simulink model "APSA"  (R2014b)
settings: Solver=FixedStepDiscrete  StartTime=0.0  StopTime=180  FixedStep=0.01  RelTol=1e-3
PreLoadFcn:
  | if exist('tl_preloadfcn','file'), tl_preloadfcn(gcs,400); end
PostLoadFcn:
  | if exist('tl_postloadfcn','file'), tl_postloadfcn(gcs,400); end
InitFcn:
  | if exist('tlds_init','file'), tlds_init(gcs); end
StartFcn:
  | if exist('tlds_start','file'), tlds_start(gcs); end
StopFcn:
  | if exist('tlds_stop','file'), tlds_stop(gcs); end
values from neighbouring files (symbols this model uses):
  EERAM_Map_Backward_Values = EERAM_Current_Map_Backward.signals.values(row,:)    [Create_Map.m]    (also in EERAM_Map_Backward_Values_2.mat = [0 0 0 0 0 0 150 150 150 150 150 150 ... (100 elements, 1x10)
  EERAM_Map_Forward_Values = EERAM_Current_Map_Forward.signals.values(row,:)    [Create_Map.m]    (also in EERAM_Map_Forward_Values_2.mat = [150 150 150 150 150 150 150 150 150 150 150 150 ... (100 el)
undefined symbols (not defined in the file or in its folder): sigbuilder_block
libraries: tllib x2
(part 2 of 3)

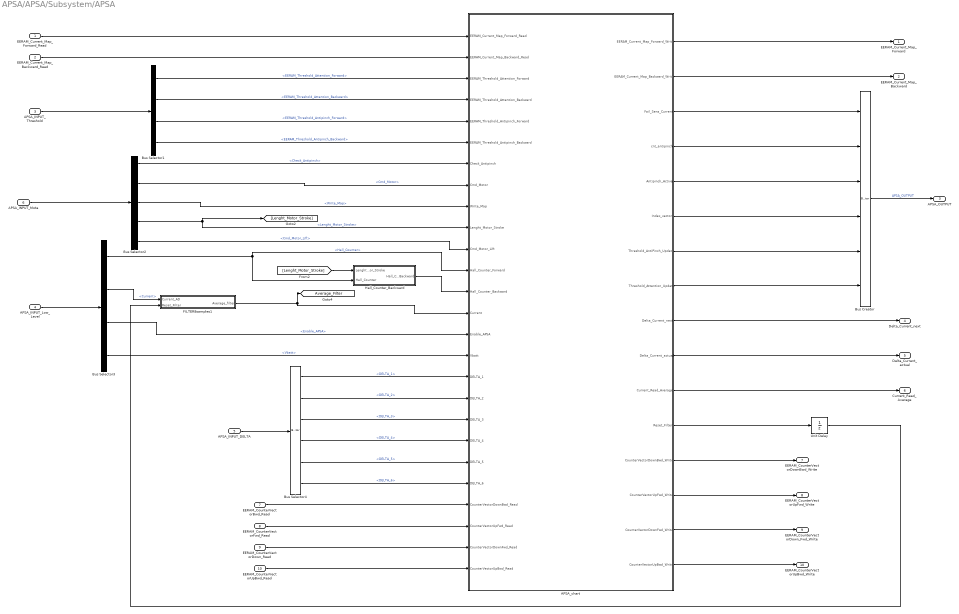
== system APSA/APSA/Subsystem/APSA ==
  EERAM_Current_Map_Forward_Read : Inport  PortDimensions=100  mask(TL_Inport){data={'output',{'variable','EERAM_Current_Map_Forward'},'date',736223.65085809026}}
      settings: DeleteFcn=if exist('delete_tlblock','file')==2,delete_tlblock(gcbh);end  OpenFcn=if exist('tl_open_blockdlg','file')==2,tl_open_blockdlg(gcbh);else,open_system(gcbh,'parameter');end
      settings: CopyFcn=|
      | if exist('tl_reset_reviewflag','file')==2
      |     tl_reset_reviewflag(gcbh);
      | end
      | if exist('tl_check_ports','file')
      |     tl_check_ports(gcbh);
      | end
      settings: NameChangeFcn=|
      | if exist('rename_tlblock','file')==2,rename_tlblock(gcbh);end
      | if exist('tl_check_ports','file'), tl_check_ports(gcbh); end
      mask Help: eval(['if exist(''tl_online_help'',''file'') == 2, tl_online_help(''Topic'',''TL_Inport''),else, web([''jar:file:///'',matlabroot,''/help/toolbox/simulink/help.jar!/slref/' lower(get_param(gcbh,'Blocktype')) '.html''], ''-helpbrowser''),end'])
      mask Display: plot([0.2 0.35 NaN 0.65 0.8],[0 1 NaN 0 1]);
  EERAM_Current_Map_Backward_Read : Inport  Port=2  PortDimensions=100  mask(TL_Inport){data={'output',{'variable','EERAM_Current_Map_Backward'},'date',736223.65094585647}}
      settings: DeleteFcn=if exist('delete_tlblock','file')==2,delete_tlblock(gcbh);end  OpenFcn=if exist('tl_open_blockdlg','file')==2,tl_open_blockdlg(gcbh);else,open_system(gcbh,'parameter');end
      settings: CopyFcn=|
      | if exist('tl_reset_reviewflag','file')==2
      |     tl_reset_reviewflag(gcbh);
      | end
      | if exist('tl_check_ports','file')
      |     tl_check_ports(gcbh);
      | end
      settings: NameChangeFcn=|
      | if exist('rename_tlblock','file')==2,rename_tlblock(gcbh);end
      | if exist('tl_check_ports','file'), tl_check_ports(gcbh); end
      mask Help: eval(['if exist(''tl_online_help'',''file'') == 2, tl_online_help(''Topic'',''TL_Inport''),else, web([''jar:file:///'',matlabroot,''/help/toolbox/simulink/help.jar!/slref/' lower(get_param(gcbh,'Blocktype')) '.html''], ''-helpbrowser''),end'])
      mask Display: plot([0.2 0.35 NaN 0.65 0.8],[0 1 NaN 0 1]);
  APSA_INPUT_Threshold : Inport  Port=3  mask(TL_BusInport){data={'#autoscaling',4,'#message',4,'#output',4,'#logdata',4,'output#1',{'variable','EERAM_Threshold_Att_Forward'},'output#2',{'variable','EERAM_Threshold_Att_Backward'},'output#3',{'variable','EERAM_Threshold_Antipinch_Forward'},'output#4',{'variable','EERAM_Threshold_Antipinch_Backward'},'signals',{{'APSA_INPUT_Threshold',{'EERAM_Threshold_Attention_Forward';'EERAM_Threshold_Attention_Backward';'EERAM_Threshold_Antipinch_Forward';'EERAM_Threshold_Antipinch_Backward'}}},'date',736307.73504877312}}
      settings: DeleteFcn=if exist('delete_tlblock','file')==2,delete_tlblock(gcbh);end  OpenFcn=if exist('tl_open_blockdlg','file')==2,tl_open_blockdlg(gcbh);else,open_system(gcbh,'parameter');end
      settings: CopyFcn=|
      | if exist('tl_reset_reviewflag','file')==2
      |     tl_reset_reviewflag(gcbh);
      | end
      | if exist('tl_check_ports','file')
      |     tl_check_ports(gcbh);
      | end
      settings: NameChangeFcn=|
      | if exist('rename_tlblock','file')==2,rename_tlblock(gcbh);end
      | if exist('tl_check_ports','file'), tl_check_ports(gcbh); end
      mask Help: eval(['if exist(''tl_online_help'',''file'') == 2, tl_online_help(''Topic'',''TL_Inport''),else, web([''jar:file:///'',matlabroot,''/help/toolbox/simulink/help.jar!/slref/' lower(get_param(gcbh,'Blocktype')) '.html''], ''-helpbrowser''),end'])
      mask Display: plot([0.2 0.35 NaN 0.65 0.8],[0 1 NaN 0 1]);
  APSA_INPUT_Low_Level : Inport  Port=4  mask(TL_BusInport){data={'#autoscaling',4,'#message',4,'#output',4,'#logdata',4,'output#1',{'name','$L','max',10000,'min',-10000},'output#2',{'name','$L','type','UInt16'},'output#3',{'name','$L','type','UInt8'},'output#4',{'name','$L'},'structvar',{'type','IMPLICIT_STRUCT','name','$L'},'signals',{{'APSA_INPUT_Low_Level',{'Hall_Counter';'Current';'Enable_APSA';'Vbatt'}}},'date',736393.5789320023}}
      settings: DeleteFcn=if exist('delete_tlblock','file')==2,delete_tlblock(gcbh);end  OpenFcn=if exist('tl_open_blockdlg','file')==2,tl_open_blockdlg(gcbh);else,open_system(gcbh,'parameter');end
      settings: CopyFcn=|
      | if exist('tl_reset_reviewflag','file')==2
      |     tl_reset_reviewflag(gcbh);
      | end
      | if exist('tl_check_ports','file')
      |     tl_check_ports(gcbh);
      | end
      settings: NameChangeFcn=|
      | if exist('rename_tlblock','file')==2,rename_tlblock(gcbh);end
      | if exist('tl_check_ports','file'), tl_check_ports(gcbh); end
      mask Help: eval(['if exist(''tl_online_help'',''file'') == 2, tl_online_help(''Topic'',''TL_Inport''),else, web([''jar:file:///'',matlabroot,''/help/toolbox/simulink/help.jar!/slref/' lower(get_param(gcbh,'Blocktype')) '.html''], ''-helpbrowser''),end'])
      mask Display: plot([0.2 0.35 NaN 0.65 0.8],[0 1 NaN 0 1]);
  APSA_INPUT_DELTA : Inport  Port=5  mask(TL_BusInport){data={'#autoscaling',6,'#message',6,'#output',6,'#logdata',6,'output#1',{'name','$L','min',0,'type','UInt8'},'output#2',{'name','$L','min',0,'type','UInt8'},'output#3',{'name','$L','min',0,'type','UInt8'},'output#4',{'name','$L','min',0,'type','UInt8'},'output#5',{'name','$L','type','UInt8'},'output#6',{'name','$L','type','UInt8'},'structvar',{'type','IMPLICIT_STRUCT','name','$L'},'signals',{{'APSA_INPUT_DELTA',{'DELTA_1';'DELTA_2';'DELTA_3';'DELTA_4';'DELTA_5';'DELTA_6'}}},'date',736307.735760162}}
      settings: DeleteFcn=if exist('delete_tlblock','file')==2,delete_tlblock(gcbh);end  OpenFcn=if exist('tl_open_blockdlg','file')==2,tl_open_blockdlg(gcbh);else,open_system(gcbh,'parameter');end
      settings: CopyFcn=|
      | if exist('tl_reset_reviewflag','file')==2
      |     tl_reset_reviewflag(gcbh);
      | end
      | if exist('tl_check_ports','file')
      |     tl_check_ports(gcbh);
      | end
      settings: NameChangeFcn=|
      | if exist('rename_tlblock','file')==2,rename_tlblock(gcbh);end
      | if exist('tl_check_ports','file'), tl_check_ports(gcbh); end
      mask Help: eval(['if exist(''tl_online_help'',''file'') == 2, tl_online_help(''Topic'',''TL_Inport''),else, web([''jar:file:///'',matlabroot,''/help/toolbox/simulink/help.jar!/slref/' lower(get_param(gcbh,'Blocktype')) '.html''], ''-helpbrowser''),end'])
      mask Display: plot([0.2 0.35 NaN 0.65 0.8],[0 1 NaN 0 1]);
  APSA_INPUT_Mota : Inport  Port=6  mask(TL_BusInport){data={'#autoscaling',5,'#message',5,'#output',5,'#logdata',5,'output#1',{'name','$L','type','UInt8'},'output#2',{'name','$L','type','UInt8'},'output#3',{'name','$L','type','UInt8'},'output#4',{'name','$L','max',5000,'min',0,'type','UInt16'},'output#5',{'name','$L','type','UInt8'},'structvar',{'type','IMPLICIT_STRUCT','name','$L'},'signals',{{'APSA_INPUT_Mota',{'Cmd_Motor';'Write_Map';'Check_Antipinch';'Lenght_Motor_Stroke';'Cmd_Motor_Lift'}}},'date',736393.58703908569}}
      settings: DeleteFcn=if exist('delete_tlblock','file')==2,delete_tlblock(gcbh);end  OpenFcn=if exist('tl_open_blockdlg','file')==2,tl_open_blockdlg(gcbh);else,open_system(gcbh,'parameter');end
      settings: CopyFcn=|
      | if exist('tl_reset_reviewflag','file')==2
      |     tl_reset_reviewflag(gcbh);
      | end
      | if exist('tl_check_ports','file')
      |     tl_check_ports(gcbh);
      | end
      settings: NameChangeFcn=|
      | if exist('rename_tlblock','file')==2,rename_tlblock(gcbh);end
      | if exist('tl_check_ports','file'), tl_check_ports(gcbh); end
      mask Help: eval(['if exist(''tl_online_help'',''file'') == 2, tl_online_help(''Topic'',''TL_Inport''),else, web([''jar:file:///'',matlabroot,''/help/toolbox/simulink/help.jar!/slref/' lower(get_param(gcbh,'Blocktype')) '.html''], ''-helpbrowser''),end'])
      mask Display: plot([0.2 0.35 NaN 0.65 0.8],[0 1 NaN 0 1]);
  EERAM_CounterVectorBwd_Read : Inport  Port=7  PortDimensions=13  mask(TL_Inport){data={'output',{'variable','EERAM_CounterVectorDownBwd'},'date',736349.65360806708}}
      settings: DeleteFcn=if exist('delete_tlblock','file')==2,delete_tlblock(gcbh);end  OpenFcn=if exist('tl_open_blockdlg','file')==2,tl_open_blockdlg(gcbh);else,open_system(gcbh,'parameter');end
      settings: CopyFcn=|
      | if exist('tl_reset_reviewflag','file')==2
      |     tl_reset_reviewflag(gcbh);
      | end
      | if exist('tl_check_ports','file')
      |     tl_check_ports(gcbh);
      | end
      settings: NameChangeFcn=|
      | if exist('rename_tlblock','file')==2,rename_tlblock(gcbh);end
      | if exist('tl_check_ports','file'), tl_check_ports(gcbh); end
      mask Help: eval(['if exist(''tl_online_help'',''file'') == 2, tl_online_help(''Topic'',''TL_Inport''),else, web([''jar:file:///'',matlabroot,''/help/toolbox/simulink/help.jar!/slref/' lower(get_param(gcbh,'Blocktype')) '.html''], ''-helpbrowser''),end'])
      mask Display: plot([0.2 0.35 NaN 0.65 0.8],[0 1 NaN 0 1]);
  EERAM_CounterVectorFwd_Read : Inport  Port=8  PortDimensions=13  mask(TL_Inport){data={'output',{'variable','EERAM_CounterVectorUpFwd'},'date',736349.65366483794}}
      settings: DeleteFcn=if exist('delete_tlblock','file')==2,delete_tlblock(gcbh);end  OpenFcn=if exist('tl_open_blockdlg','file')==2,tl_open_blockdlg(gcbh);else,open_system(gcbh,'parameter');end
      settings: CopyFcn=|
      | if exist('tl_reset_reviewflag','file')==2
      |     tl_reset_reviewflag(gcbh);
      | end
      | if exist('tl_check_ports','file')
      |     tl_check_ports(gcbh);
      | end
      settings: NameChangeFcn=|
      | if exist('rename_tlblock','file')==2,rename_tlblock(gcbh);end
      | if exist('tl_check_ports','file'), tl_check_ports(gcbh); end
      mask Help: eval(['if exist(''tl_online_help'',''file'') == 2, tl_online_help(''Topic'',''TL_Inport''),else, web([''jar:file:///'',matlabroot,''/help/toolbox/simulink/help.jar!/slref/' lower(get_param(gcbh,'Blocktype')) '.html''], ''-helpbrowser''),end'])
      mask Display: plot([0.2 0.35 NaN 0.65 0.8],[0 1 NaN 0 1]);
  EERAM_CounterVectorDown_Read : Inport  Port=9  PortDimensions=13  mask(TL_Inport){data={'output',{'variable','EERAM_CounterVectorDownFwd'},'date',736349.6566348843}}
      settings: DeleteFcn=if exist('delete_tlblock','file')==2,delete_tlblock(gcbh);end  OpenFcn=if exist('tl_open_blockdlg','file')==2,tl_open_blockdlg(gcbh);else,open_system(gcbh,'parameter');end
      settings: CopyFcn=|
      | if exist('tl_reset_reviewflag','file')==2
      |     tl_reset_reviewflag(gcbh);
      | end
      | if exist('tl_check_ports','file')
      |     tl_check_ports(gcbh);
      | end
      settings: NameChangeFcn=|
      | if exist('rename_tlblock','file')==2,rename_tlblock(gcbh);end
      | if exist('tl_check_ports','file'), tl_check_ports(gcbh); end
      mask Help: eval(['if exist(''tl_online_help'',''file'') == 2, tl_online_help(''Topic'',''TL_Inport''),else, web([''jar:file:///'',matlabroot,''/help/toolbox/simulink/help.jar!/slref/' lower(get_param(gcbh,'Blocktype')) '.html''], ''-helpbrowser''),end'])
      mask Display: plot([0.2 0.35 NaN 0.65 0.8],[0 1 NaN 0 1]);
  EERAM_CounterVectorUpBwd_Read : Inport  Port=10  PortDimensions=13  mask(TL_Inport){data={'output',{'variable','EERAM_CounterVectorUpBwd'},'date',736349.6567374653}}
      settings: DeleteFcn=if exist('delete_tlblock','file')==2,delete_tlblock(gcbh);end  OpenFcn=if exist('tl_open_blockdlg','file')==2,tl_open_blockdlg(gcbh);else,open_system(gcbh,'parameter');end
      settings: CopyFcn=|
      | if exist('tl_reset_reviewflag','file')==2
      |     tl_reset_reviewflag(gcbh);
      | end
      | if exist('tl_check_ports','file')
      |     tl_check_ports(gcbh);
      | end
      settings: NameChangeFcn=|
      | if exist('rename_tlblock','file')==2,rename_tlblock(gcbh);end
      | if exist('tl_check_ports','file'), tl_check_ports(gcbh); end
      mask Help: eval(['if exist(''tl_online_help'',''file'') == 2, tl_online_help(''Topic'',''TL_Inport''),else, web([''jar:file:///'',matlabroot,''/help/toolbox/simulink/help.jar!/slref/' lower(get_param(gcbh,'Blocktype')) '.html''], ''-helpbrowser''),end'])
      mask Display: plot([0.2 0.35 NaN 0.65 0.8],[0 1 NaN 0 1]);
  APSA_chart : Stateflow chart  TreatAsAtomicUnit=on
  Bus Creator : BusCreator  Inputs=6
  Bus Selector1 : BusSelector  OutputSignals=EERAM_Threshold_Attention_Forward,EERAM_Threshold_Attention_Backward,EERAM_Threshold_Antipinch_Forward,EERAM_Threshold_Antipinch_Backward
  Bus Selector2 : BusSelector  OutputSignals=Check_Antipinch,Cmd_Motor,Write_Map,Lenght_Motor_Stroke,Cmd_Motor_Lift
  Bus Selector3 : BusSelector  OutputSignals=Hall_Counter,Current,Enable_APSA,Vbatt
  Bus Selector4 : BusSelector  OutputSignals=DELTA_1,DELTA_2,DELTA_3,DELTA_4,DELTA_5,DELTA_6
  FILTER8samples1 : Subsystem
  Hall_Counter_Backward : Subsystem
  Unit Delay : UnitDelay  SampleTime=-1  mask(TL_UnitDelay){data={'output',{'type','UInt8'},'state',{'type','UInt8'},'date',736291.48166902782}}
      settings: CopyFcn=if exist('tl_reset_reviewflag') == 2, tl_reset_reviewflag(gcbh); end  DeleteFcn=if exist('delete_tlblock','file')==2,delete_tlblock(gcbh);end  NameChangeFcn=if exist('rename_tlblock','file')==2,rename_tlblock(gcbh);end  OpenFcn=if exist('tl_open_blockdlg','file')==2,tl_open_blockdlg(gcbh);else,open_system(gcbh,'parameter');end
      mask Help: eval(['if exist(''tl_online_help'',''file'') == 2, tl_online_help(''Topic'',''TL_UnitDelay''),else, web([''jar:file:///'',matlabroot,''/help/toolbox/simulink/help.jar!/slref/' lower(get_param(gcbh,'Blocktype')) '.html''], ''-helpbrowser''),end'])
      mask Display: plot([-0.1, 1.05, NaN, -0.1, 1.05],[.01, .01, NaN, .99, .99]);
  EERAM_Current_Map_Forward : Outport  PortDimensions=100  mask(TL_Outport){data={'output',{'variable','EERAM_Current_Map_Forward'},'date',736223.65313251154}}
      settings: DeleteFcn=if exist('delete_tlblock','file')==2,delete_tlblock(gcbh);end  OpenFcn=if exist('tl_open_blockdlg','file')==2,tl_open_blockdlg(gcbh);else,open_system(gcbh,'parameter');end
      settings: CopyFcn=|
      | if exist('tl_reset_reviewflag','file')==2
      |     tl_reset_reviewflag(gcbh);
      | end
      | if exist('tl_check_ports','file')
      |     tl_check_ports(gcbh);
      | end
      settings: NameChangeFcn=|
      | if exist('rename_tlblock','file')==2,rename_tlblock(gcbh);end
      | if exist('tl_check_ports','file'), tl_check_ports(gcbh); end
      mask Help: eval(['if exist(''tl_online_help'',''file'') == 2, tl_online_help(''Topic'',''TL_Outport''),else, web([''jar:file:///'',matlabroot,''/help/toolbox/simulink/help.jar!/slref/' lower(get_param(gcbh,'Blocktype')) '.html''], ''-helpbrowser''),end'])
      mask Display: plot([0.2 0.35 NaN 0.65 0.8],[0 1 NaN 0 1]);
  EERAM_Current_Map_Backward : Outport  Port=2  PortDimensions=100  mask(TL_Outport){data={'output',{'variable','EERAM_Current_Map_Backward'},'date',736223.65323016199}}
      settings: DeleteFcn=if exist('delete_tlblock','file')==2,delete_tlblock(gcbh);end  OpenFcn=if exist('tl_open_blockdlg','file')==2,tl_open_blockdlg(gcbh);else,open_system(gcbh,'parameter');end
      settings: CopyFcn=|
      | if exist('tl_reset_reviewflag','file')==2
      |     tl_reset_reviewflag(gcbh);
      | end
      | if exist('tl_check_ports','file')
      |     tl_check_ports(gcbh);
      | end
      settings: NameChangeFcn=|
      | if exist('rename_tlblock','file')==2,rename_tlblock(gcbh);end
      | if exist('tl_check_ports','file'), tl_check_ports(gcbh); end
      mask Help: eval(['if exist(''tl_online_help'',''file'') == 2, tl_online_help(''Topic'',''TL_Outport''),else, web([''jar:file:///'',matlabroot,''/help/toolbox/simulink/help.jar!/slref/' lower(get_param(gcbh,'Blocktype')) '.html''], ''-helpbrowser''),end'])
      mask Display: plot([0.2 0.35 NaN 0.65 0.8],[0 1 NaN 0 1]);
  APSA_OUTPUT : Outport  Port=3  mask(TL_BusOutport){data={'#autoscaling',6,'#message',6,'#output',6,'#logdata',6,'output#1',{'variable','Fail_Sens_Current'},'output#2',{'name','$L'},'output#3',{'variable','Antipinch_Active'},'output#4',{'variable','Index_vector'},'output#5',{'variable','Threshold_AntiPinch_Update'},'output#6',{'variable','Threshold_Attention_Update'},'structvar',{'type','IMPLICIT_STRUCT','name','$L'},'signals',{{'APSA_OUTPUT',{'Fail_Sens_Current';'cnt_antipinch';'Antipinch_Active';'Index_vector';'Threshold_AntiPinch_Update';'Threshold_Attention_Update'}}},'date',736307.74256392359}}
      settings: DeleteFcn=if exist('delete_tlblock','file')==2,delete_tlblock(gcbh);end  OpenFcn=if exist('tl_open_blockdlg','file')==2,tl_open_blockdlg(gcbh);else,open_system(gcbh,'parameter');end
      settings: CopyFcn=|
      | if exist('tl_reset_reviewflag','file')==2
      |     tl_reset_reviewflag(gcbh);
      | end
      | if exist('tl_check_ports','file')
      |     tl_check_ports(gcbh);
      | end
      settings: NameChangeFcn=|
      | if exist('rename_tlblock','file')==2,rename_tlblock(gcbh);end
      | if exist('tl_check_ports','file'), tl_check_ports(gcbh); end
      mask Help: eval(['if exist(''tl_online_help'',''file'') == 2, tl_online_help(''Topic'',''TL_Outport''),else, web([''jar:file:///'',matlabroot,''/help/toolbox/simulink/help.jar!/slref/' lower(get_param(gcbh,'Blocktype')) '.html''], ''-helpbrowser''),end'])
      mask Display: plot([0.2 0.35 NaN 0.65 0.8],[0 1 NaN 0 1]);
  Delta_Current_next : Outport  Port=4  mask(TL_Outport){data={'output',{'name','Delta_Current_next'},'date',736293.39429296297}}
      settings: DeleteFcn=if exist('delete_tlblock','file')==2,delete_tlblock(gcbh);end  OpenFcn=if exist('tl_open_blockdlg','file')==2,tl_open_blockdlg(gcbh);else,open_system(gcbh,'parameter');end
      settings: CopyFcn=|
      | if exist('tl_reset_reviewflag','file')==2
      |     tl_reset_reviewflag(gcbh);
      | end
      | if exist('tl_check_ports','file')
      |     tl_check_ports(gcbh);
      | end
      settings: NameChangeFcn=|
      | if exist('rename_tlblock','file')==2,rename_tlblock(gcbh);end
      | if exist('tl_check_ports','file'), tl_check_ports(gcbh); end
      mask Help: eval(['if exist(''tl_online_help'',''file'') == 2, tl_online_help(''Topic'',''TL_Outport''),else, web([''jar:file:///'',matlabroot,''/help/toolbox/simulink/help.jar!/slref/' lower(get_param(gcbh,'Blocktype')) '.html''], ''-helpbrowser''),end'])
      mask Display: plot([0.2 0.35 NaN 0.65 0.8],[0 1 NaN 0 1]);
  Delta_Current_actual : Outport  Port=5  mask(TL_Outport){data={'output',{'name','Delta_Current_actual'},'date',736293.39420129627}}
      settings: DeleteFcn=if exist('delete_tlblock','file')==2,delete_tlblock(gcbh);end  OpenFcn=if exist('tl_open_blockdlg','file')==2,tl_open_blockdlg(gcbh);else,open_system(gcbh,'parameter');end
      settings: CopyFcn=|
      | if exist('tl_reset_reviewflag','file')==2
      |     tl_reset_reviewflag(gcbh);
      | end
      | if exist('tl_check_ports','file')
      |     tl_check_ports(gcbh);
      | end
      settings: NameChangeFcn=|
      | if exist('rename_tlblock','file')==2,rename_tlblock(gcbh);end
      | if exist('tl_check_ports','file'), tl_check_ports(gcbh); end
      mask Help: eval(['if exist(''tl_online_help'',''file'') == 2, tl_online_help(''Topic'',''TL_Outport''),else, web([''jar:file:///'',matlabroot,''/help/toolbox/simulink/help.jar!/slref/' lower(get_param(gcbh,'Blocktype')) '.html''], ''-helpbrowser''),end'])
      mask Display: plot([0.2 0.35 NaN 0.65 0.8],[0 1 NaN 0 1]);
  Current_Read_Average : Outport  Port=6  mask(TL_Outport){data={'output',{'name','Current_Read_Average'},'date',736245.42948233802}}
      settings: DeleteFcn=if exist('delete_tlblock','file')==2,delete_tlblock(gcbh);end  OpenFcn=if exist('tl_open_blockdlg','file')==2,tl_open_blockdlg(gcbh);else,open_system(gcbh,'parameter');end
      settings: CopyFcn=|
      | if exist('tl_reset_reviewflag','file')==2
      |     tl_reset_reviewflag(gcbh);
      | end
      | if exist('tl_check_ports','file')
      |     tl_check_ports(gcbh);
      | end
      settings: NameChangeFcn=|
      | if exist('rename_tlblock','file')==2,rename_tlblock(gcbh);end
      | if exist('tl_check_ports','file'), tl_check_ports(gcbh); end
      mask Help: eval(['if exist(''tl_online_help'',''file'') == 2, tl_online_help(''Topic'',''TL_Outport''),else, web([''jar:file:///'',matlabroot,''/help/toolbox/simulink/help.jar!/slref/' lower(get_param(gcbh,'Blocktype')) '.html''], ''-helpbrowser''),end'])
      mask Display: plot([0.2 0.35 NaN 0.65 0.8],[0 1 NaN 0 1]);
  EERAM_CounterVectorDownBwd_Write : Outport  Port=7  PortDimensions=13  mask(TL_Outport){data={'output',{'variable','EERAM_CounterVectorDownBwd'},'date',736349.653609375}}
      settings: DeleteFcn=if exist('delete_tlblock','file')==2,delete_tlblock(gcbh);end  OpenFcn=if exist('tl_open_blockdlg','file')==2,tl_open_blockdlg(gcbh);else,open_system(gcbh,'parameter');end
      settings: CopyFcn=|
      | if exist('tl_reset_reviewflag','file')==2
      |     tl_reset_reviewflag(gcbh);
      | end
      | if exist('tl_check_ports','file')
      |     tl_check_ports(gcbh);
      | end
      settings: NameChangeFcn=|
      | if exist('rename_tlblock','file')==2,rename_tlblock(gcbh);end
      | if exist('tl_check_ports','file'), tl_check_ports(gcbh); end
      mask Help: eval(['if exist(''tl_online_help'',''file'') == 2, tl_online_help(''Topic'',''TL_Outport''),else, web([''jar:file:///'',matlabroot,''/help/toolbox/simulink/help.jar!/slref/' lower(get_param(gcbh,'Blocktype')) '.html''], ''-helpbrowser''),end'])
      mask Display: plot([0.2 0.35 NaN 0.65 0.8],[0 1 NaN 0 1]);
  EERAM_CounterVectorUpFwd_Write : Outport  Port=8  PortDimensions=13  mask(TL_Outport){data={'output',{'variable','EERAM_CounterVectorUpFwd'},'date',736349.65366504632}}
      settings: DeleteFcn=if exist('delete_tlblock','file')==2,delete_tlblock(gcbh);end  OpenFcn=if exist('tl_open_blockdlg','file')==2,tl_open_blockdlg(gcbh);else,open_system(gcbh,'parameter');end
      settings: CopyFcn=|
      | if exist('tl_reset_reviewflag','file')==2
      |     tl_reset_reviewflag(gcbh);
      | end
      | if exist('tl_check_ports','file')
      |     tl_check_ports(gcbh);
      | end
      settings: NameChangeFcn=|
      | if exist('rename_tlblock','file')==2,rename_tlblock(gcbh);end
      | if exist('tl_check_ports','file'), tl_check_ports(gcbh); end
      mask Help: eval(['if exist(''tl_online_help'',''file'') == 2, tl_online_help(''Topic'',''TL_Outport''),else, web([''jar:file:///'',matlabroot,''/help/toolbox/simulink/help.jar!/slref/' lower(get_param(gcbh,'Blocktype')) '.html''], ''-helpbrowser''),end'])
      mask Display: plot([0.2 0.35 NaN 0.65 0.8],[0 1 NaN 0 1]);
  EERAM_CounterVectorDown_Fwd_Write : Outport  Port=9  PortDimensions=13  mask(TL_Outport){data={'output',{'variable','EERAM_CounterVectorDownFwd'},'date',736349.65545192128}}
      settings: DeleteFcn=if exist('delete_tlblock','file')==2,delete_tlblock(gcbh);end  OpenFcn=if exist('tl_open_blockdlg','file')==2,tl_open_blockdlg(gcbh);else,open_system(gcbh,'parameter');end
      settings: CopyFcn=|
      | if exist('tl_reset_reviewflag','file')==2
      |     tl_reset_reviewflag(gcbh);
      | end
      | if exist('tl_check_ports','file')
      |     tl_check_ports(gcbh);
      | end
      settings: NameChangeFcn=|
      | if exist('rename_tlblock','file')==2,rename_tlblock(gcbh);end
      | if exist('tl_check_ports','file'), tl_check_ports(gcbh); end
      mask Help: eval(['if exist(''tl_online_help'',''file'') == 2, tl_online_help(''Topic'',''TL_Outport''),else, web([''jar:file:///'',matlabroot,''/help/toolbox/simulink/help.jar!/slref/' lower(get_param(gcbh,'Blocktype')) '.html''], ''-helpbrowser''),end'])
      mask Display: plot([0.2 0.35 NaN 0.65 0.8],[0 1 NaN 0 1]);
  EERAM_CounterVectorUpBwd_Write : Outport  Port=10  PortDimensions=13  mask(TL_Outport){data={'output',{'variable','EERAM_CounterVectorUpBwd'},'date',736349.6557187268}}
      settings: DeleteFcn=if exist('delete_tlblock','file')==2,delete_tlblock(gcbh);end  OpenFcn=if exist('tl_open_blockdlg','file')==2,tl_open_blockdlg(gcbh);else,open_system(gcbh,'parameter');end
      settings: CopyFcn=|
      | if exist('tl_reset_reviewflag','file')==2
      |     tl_reset_reviewflag(gcbh);
      | end
      | if exist('tl_check_ports','file')
      |     tl_check_ports(gcbh);
      | end
      settings: NameChangeFcn=|
      | if exist('rename_tlblock','file')==2,rename_tlblock(gcbh);end
      | if exist('tl_check_ports','file'), tl_check_ports(gcbh); end
      mask Help: eval(['if exist(''tl_online_help'',''file'') == 2, tl_online_help(''Topic'',''TL_Outport''),else, web([''jar:file:///'',matlabroot,''/help/toolbox/simulink/help.jar!/slref/' lower(get_param(gcbh,'Blocktype')) '.html''], ''-helpbrowser''),end'])
      mask Display: plot([0.2 0.35 NaN 0.65 0.8],[0 1 NaN 0 1]);
  tag scope: Average_Filter=global
  wires:
  APSA_INPUT_Threshold/1 -> Bus Selector1/1
  APSA_INPUT_Mota/1 -> Bus Selector2/1
  APSA_INPUT_Low_Level/1 -> Bus Selector3/1
  Bus Selector1/3 -> APSA_chart/5(EERAM_Threshold_Antipinch_Forward)  "<EERAM_Threshold_Antipinch_Forward>"
  Bus Selector2/1 -> APSA_chart/7(Check_Antipinch)  "<Check_Antipinch>"
  Bus Selector2/3 -> APSA_chart/9(Write_Map)  "<Write_Map>"
  Bus Selector2/4 -> [Lenght_Motor_Stroke], APSA_chart/10(Lenght_Motor_Stroke)  "<Lenght_Motor_Stroke>"
  Bus Selector3/1 -> APSA_chart/12(Hall_Counter_Forward), Hall_Counter_Backward/2(Hall_Counter)  "<Hall_Counter>"
  APSA_chart/1(EERAM_Current_Map_Forward_Write) -> EERAM_Current_Map_Forward/1
  Bus Selector2/2 -> APSA_chart/8(Cmd_Motor)  "<Cmd_Motor>"
  EERAM_Current_Map_Forward_Read/1 -> APSA_chart/1(EERAM_Current_Map_Forward_Read)
  Bus Selector1/1 -> APSA_chart/3(EERAM_Threshold_Attention_Forward)  "<EERAM_Threshold_Attention_Forward>"
  APSA_INPUT_DELTA/1 -> Bus Selector4/1
  Bus Selector4/1 -> APSA_chart/17(DELTA_1)  "<DELTA_1>"
  Bus Selector4/2 -> APSA_chart/18(DELTA_2)  "<DELTA_2>"
  Bus Selector4/3 -> APSA_chart/19(DELTA_3)  "<DELTA_3>"
  Bus Selector4/4 -> APSA_chart/20(DELTA_4)  "<DELTA_4>"
  Bus Selector4/5 -> APSA_chart/21(DELTA_5)  "<DELTA_5>"
  Bus Selector4/6 -> APSA_chart/22(DELTA_6)  "<DELTA_6>"
  Bus Selector1/2 -> APSA_chart/4(EERAM_Threshold_Attention_Backward)  "<EERAM_Threshold_Attention_Backward>"
  EERAM_Current_Map_Backward_Read/1 -> APSA_chart/2(EERAM_Current_Map_Backward_Read)
  Bus Selector3/3 -> APSA_chart/15(Enable_APSA)  "<Enable_APSA>"
  APSA_chart/10(Delta_Current_actual) -> Delta_Current_actual/1
  APSA_chart/9(Delta_Current_next) -> Delta_Current_next/1
  Bus Creator/1 -> APSA_OUTPUT/1  "APSA_OUTPUT"
  APSA_chart/11(Current_Read_Average) -> Current_Read_Average/1
  APSA_chart/3(Fail_Sens_Current) -> Bus Creator/1
  APSA_chart/4(cnt_antipinch) -> Bus Creator/2
  APSA_chart/5(Antipinch_Active) -> Bus Creator/3
  APSA_chart/6(Index_vector) -> Bus Creator/4
  APSA_chart/7(Threshold_AntiPinch_Update) -> Bus Creator/5
  APSA_chart/8(Threshold_Attention_Update) -> Bus Creator/6
  Hall_Counter_Backward/1(Hall_Counter_Backward) -> APSA_chart/13(Hall_Counter_Backward)
  Bus Selector1/4 -> APSA_chart/6(EERAM_Threshold_Antipinch_Backward)  "<EERAM_Threshold_Antipinch_Backward>"
  [Lenght_Motor_Stroke] -> Hall_Counter_Backward/1(Lenght_Motor_Stroke)
  Bus Selector3/2 -> FILTER8samples1/1(Current_AD)  "<Current>"
  FILTER8samples1/1(Average_filter) -> [Average_Filter], APSA_chart/14(Current)
  APSA_chart/2(EERAM_Current_Map_Backward_Write) -> EERAM_Current_Map_Backward/1
  APSA_chart/12(Reset_Filter) -> Unit Delay/1
  Unit Delay/1 -> FILTER8samples1/2(Reset_Filter)
  EERAM_CounterVectorBwd_Read/1 -> APSA_chart/23(CounterVectorDownBwd_Read)
  EERAM_CounterVectorFwd_Read/1 -> APSA_chart/24(CounterVectorUpFwd_Read)
  APSA_chart/13(CounterVectorDownBwd_Write) -> EERAM_CounterVectorDownBwd_Write/1
  APSA_chart/14(CounterVectorUpFwd_Write) -> EERAM_CounterVectorUpFwd_Write/1
  APSA_chart/15(CounterVectorDownFwd_Write) -> EERAM_CounterVectorDown_Fwd_Write/1
  APSA_chart/16(CounterVectorUpBwd_Write) -> EERAM_CounterVectorUpBwd_Write/1
  EERAM_CounterVectorDown_Read/1 -> APSA_chart/25(CounterVectorDownFwd_Read)
  EERAM_CounterVectorUpBwd_Read/1 -> APSA_chart/26(CounterVectorUpBwd_Read)
  Bus Selector3/4 -> APSA_chart/16(Vbatt)  "<Vbatt>"
  Bus Selector2/5 -> APSA_chart/11(Cmd_Motor_Lift)  "<Cmd_Motor_Lift>"

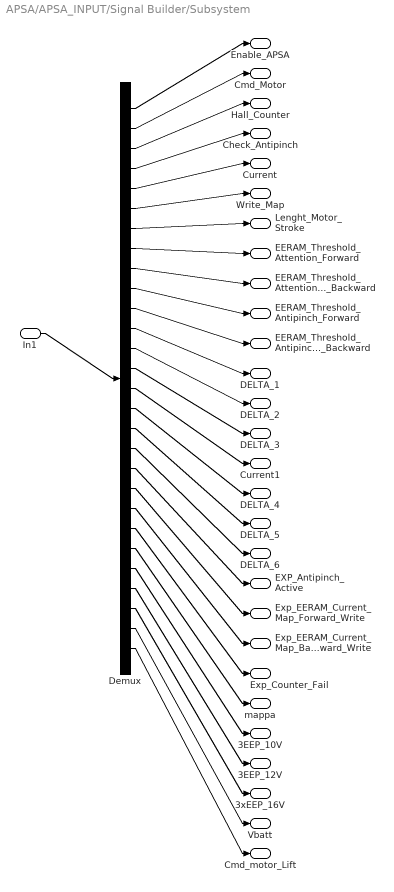
== system APSA/APSA_INPUT/Signal Builder/Subsystem ==
  In1 : Inport
  Demux : Demux  Tag=STV Demux  Outputs=28
  Enable_APSA : Outport  Tag=STV Outport
  Cmd_Motor : Outport  Tag=STV Outport  Port=2
  Hall_Counter : Outport  Tag=STV Outport  Port=3
  "Check_Antipinch " : Outport  Tag=STV Outport  Port=4
  Current : Outport  Tag=STV Outport  Port=5
  Write_Map : Outport  Tag=STV Outport  Port=6
  Lenght_Motor_Stroke : Outport  Tag=STV Outport  Port=7
  EERAM_Threshold_Attention_Forward : Outport  Tag=STV Outport  Port=8
  EERAM_Threshold_Attention_Backward : Outport  Tag=STV Outport  Port=9
  EERAM_Threshold_Antipinch_Forward : Outport  Tag=STV Outport  Port=10
  EERAM_Threshold_Antipinch_Backward : Outport  Tag=STV Outport  Port=11
  DELTA_1 : Outport  Tag=STV Outport  Port=12
  DELTA_2 : Outport  Tag=STV Outport  Port=13
  DELTA_3 : Outport  Tag=STV Outport  Port=14
  Current1 : Outport  Tag=STV Outport  Port=15
  DELTA_4 : Outport  Tag=STV Outport  Port=16
  DELTA_5 : Outport  Tag=STV Outport  Port=17
  DELTA_6 : Outport  Tag=STV Outport  Port=18
  EXP_Antipinch_Active : Outport  Tag=STV Outport  Port=19
  Exp_EERAM_Current_Map_Forward_Write : Outport  Tag=STV Outport  Port=20
  Exp_EERAM_Current_Map_Backward_Write : Outport  Tag=STV Outport  Port=21
  Exp_Counter_Fail : Outport  Tag=STV Outport  Port=22
  mappa : Outport  Tag=STV Outport  Port=23
  3EEP_10V : Outport  Tag=STV Outport  Port=24
  3EEP_12V : Outport  Tag=STV Outport  Port=25
  3xEEP_16V : Outport  Tag=STV Outport  Port=26
  Vbatt : Outport  Tag=STV Outport  Port=27
  Cmd_motor_Lift : Outport  Tag=STV Outport  Port=28
  wires:
  In1/1 -> Demux/1
  Demux/1 -> Enable_APSA/1
  Demux/2 -> Cmd_Motor/1
  Demux/3 -> Hall_Counter/1
  Demux/4 -> "Check_Antipinch "/1
  Demux/5 -> Current/1
  Demux/6 -> Write_Map/1
  Demux/7 -> Lenght_Motor_Stroke/1
  Demux/8 -> EERAM_Threshold_Attention_Forward/1
  Demux/9 -> EERAM_Threshold_Attention_Backward/1
  Demux/10 -> EERAM_Threshold_Antipinch_Forward/1
  Demux/11 -> EERAM_Threshold_Antipinch_Backward/1
  Demux/12 -> DELTA_1/1
  Demux/13 -> DELTA_2/1
  Demux/14 -> DELTA_3/1
  Demux/15 -> Current1/1
  Demux/16 -> DELTA_4/1
  Demux/17 -> DELTA_5/1
  Demux/18 -> DELTA_6/1
  Demux/19 -> EXP_Antipinch_Active/1
  Demux/20 -> Exp_EERAM_Current_Map_Forward_Write/1
  Demux/21 -> Exp_EERAM_Current_Map_Backward_Write/1
  Demux/22 -> Exp_Counter_Fail/1
  Demux/23 -> mappa/1
  Demux/24 -> 3EEP_10V/1
  Demux/25 -> 3EEP_12V/1
  Demux/26 -> 3xEEP_16V/1
  Demux/27 -> Vbatt/1
  Demux/28 -> Cmd_motor_Lift/1

== system APSA/APSA/Subsystem/APSA/FILTER8samples1 ==
  Current_AD : Inport
  Reset_Filter : Inport  Port=2
  Average_mobile_Filter_8samp : Stateflow chart  TreatAsAtomicUnit=on
  Average_filter : Outport  InitialOutput=0
  wires:
  Average_mobile_Filter_8samp/1(average_filter) -> Average_filter/1  "Average_filter"
  Current_AD/1 -> Average_mobile_Filter_8samp/1(Current_AD)
  Reset_Filter/1 -> Average_mobile_Filter_8samp/2(Reset_Filter)

== system APSA/APSA/Subsystem/APSA/Hall_Counter_Backward ==
  Lenght_Motor_Stroke : Inport  OutMin=0  OutMax=5000  OutDataTypeStr=uint16
  Hall_Counter : Inport  Port=2  OutMin=-10000  OutMax=10000  OutDataTypeStr=int16
  Sum : Sum  Inputs=+-  OutDataTypeStr=int16  mask(TL_Sum){data={'date',736298.43431873841}}
      settings: CopyFcn=if exist('tl_reset_reviewflag','file')==2,tl_reset_reviewflag(gcbh);end  DeleteFcn=if exist('delete_tlblock','file')==2,delete_tlblock(gcbh);end  NameChangeFcn=if exist('rename_tlblock','file')==2,rename_tlblock(gcbh);end  OpenFcn=if exist('tl_open_blockdlg','file')==2,tl_open_blockdlg(gcbh);else,open_system(gcbh,'parameter');end
      mask Help: eval(['if exist(''tl_online_help'',''file'') == 2, tl_online_help(''Topic'',''TL_Sum''),else, web([''jar:file:///'',matlabroot,''/help/toolbox/simulink/help.jar!/slref/' lower(get_param(gcbh,'Blocktype')) '.html''], ''-helpbrowser''),end'])
      mask Display: plot([-0.1, 1.05, NaN, -0.1, 1.05],[.01, .01, NaN, .99, .99]);
  Hall_Counter_Backward : Outport
  wires:
  Lenght_Motor_Stroke/1 -> Sum/1
  Hall_Counter/1 -> Sum/2
  Sum/1 -> Hall_Counter_Backward/1  "Hall_Counter_Backward"
